simulink model "AdmittanceScanPRBS"  (R2025a)
settings: Solver=VariableStepAuto  StartTime=0.0  StopTime=Tsim  RelTol=1e-3
PreLoadFcn:
  | SimulationTime = 10;
  | AdmittanceScanParameters;
undefined symbols (not defined in the file): Array, Base, BatteryInverter, DiscIntNeverNeededParam, ee_sli_rtmsupport, feeder, fRT, frt, gcbh, GFLBatteryController, GFMBatteryController, gGFM, grid, Grid, line, loadpq, loadstep1, loadstep2, lvrt, LVRT, mGFM, Panel, pll, pmsm, PVController, PVInverter, PVTransformer, scan, time, Ts, VSMbase, windController, windTurbine
libraries: ee_lib x19, eeGeneralControl x17, nesl_utility x16, fl_lib x10, eeTransforms x9, simulink x8, slpidlib x2, batteryecm_lib x1, simulink_extras x1, eePowerMeasurement x1
(part 1 of 4)
settings Model: SimulationMode=accelerator  PacingRate=1.100000  Creator=rajarshd  LastModifiedBy=rajarshd
settings DataIOCC: ReturnWorkspaceOutputsName=Data
settings OptimizationCC: BlockReduction=off  DefaultParameterBehavior=Inlined  BufferReuse=off
settings RTWCC: GPUComputeCapability=3.5

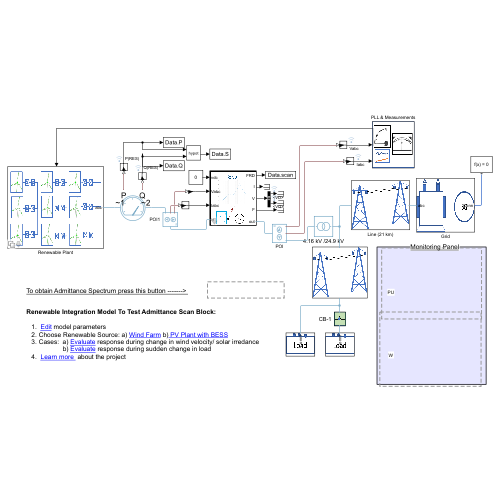
[thumbnail: Simulink's stored preview of the top-level diagram]
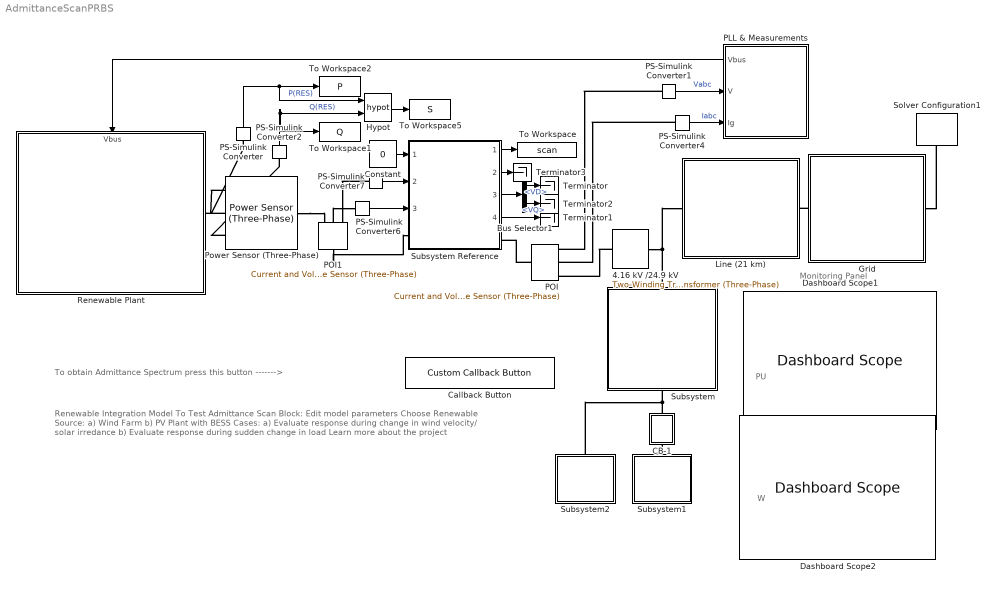
== system AdmittanceScanPRBS ==
  note: W
  note: PU
  note: Monitoring Panel
  note: To obtain Admittance Spectrum press this button ------->
  note: Renewable Integration Model To Test Admittance Scan Block:
      |
      | Edit model parameters
      | Choose Renewable Source: a) Wind Farm b) PV Plant with BESS
      | Cases: a) Evaluate response during change in wind velocity/ solar irredance
      | b) Evaluate response during sudden change in load
      | Learn more about the project
  4.16 kV /24.9 kV : ee_lib/Passive/Transformers/Two-Winding Transformer (Three-Phase)  SRated=PVTransformer.VA A*V  FRated=Grid.frequency Hz  Winding1Connection=ee.enum.windingconnection.Yg  VRated1=PVTransformer.hv V  Winding2Connection=ee.enum.windingconnection.Yg  VRated2=PVTransformer.lv V  CoreType=ee.enum.coretype.threelimb  pu_Rw1=PVTransformer.winding_resistance/2  pu_Rw2=PVTransformer.winding_resistance/2  leakage_reactance_option=ee.enum.transformer_leakage.include  pu_Xl1=PVTransformer.winding_lekage_reactance/2  pu_Xl2=PVTransformer.winding_lekage_reactance/2  magnetizing_resistance_option=ee.enum.transformer_magnetizingResistance.exclude  pu_Rm=500  magnetizing_reactance_option=ee.enum.transformer_magnetizingReactance.exclude  saturation_option=ee.enum.transformer_saturation.exclude  pu_Xm=500  current_data=[0, .002, 1, 2]  magnetic_flux_data=[0, 1.2, 1.5, 1.51]  pu_X0=PVTransformer.zero_sequence_reactance  i1_specify=off  i1_priority=None  i1=[0, 0, 0] A  i1_nominal_specify=off  i1_nominal_value=1  i1_nominal_unit=A  i2_specify=off  i2_priority=None  i2=[0, 0, 0] A  i2_nominal_specify=off  i2_nominal_value=1  i2_nominal_unit=A  phi_specify=off  phi_priority=None  phi=[0, 0, 0]  phi_nominal_specify=off  phi_nominal_value=1  phi_nominal_unit=1  power_dissipated_specify=off  power_dissipated_priority=None  power_dissipated=0 W  power_dissipated_nominal_specify=off  power_dissipated_nominal_value=1  power_dissipated_nominal_unit=W
      settings: InternalSimscapePortConfiguration="{\"Bottom\":[],\"Left\":[{\"id\":\"N1\",\"label\":\"~1\",\"type\":\"foundation.electrical.three_phase\"}],\"Right\":[{\"id\":\"N2\",\"label\":\"~2\",\"type\":\"foundation.electrical.three_phase\"}],\"Top\":[]}"
  Bus Selector1 : BusSelector  OutputSignals=VD,VQ
  CB-1 : Subsystem
      mask Display: image('$imagefile'); % Use "Edit Image" on toolstrip to change.
  Callback Button : CustomCallbackButton  Configuration="{\"components\":[{\"name\":\"BackgroundImageComponent\",\"settings\":{\"image\":{\"size\":[0,0],\"src\":\"default\",\"srcOrientation\":\"Right\"},\"position\":[0,0,1,1]}},{\"name\":\"ButtonStateComponent\",\"settings\":{\"buttonType\":\"latch\",\"clickFcn\":\"Data=sim(bdroot);\\nadmittancescanPRBS(scan.Vd,scan.Vq,scan.Vdc,scan.f,Data.scan,modelorder) \",\"latched\":false,\"offValue\":null,\"onValue\":1,\"position\":[0,0,1,1],\"pressDelay\":\"500\",\"pressFcn\":\"\",\"repeatInterval\":\"0\",\"states\":[{\"horizontalAlignment\":\"center\",\"image\":{\"position\":[0,0,1,1],\"size\":[1,1],\"src\":\"default\",\"srcOrientation\":\"Right\"},\"label\":{\"color\":[1,1,1],\"icon\":{\"size\":[0,0],\"src\":\"default\",\"srcOrientation\":\"Right\"},\"iconOffset\":0,\"iconPlacement\":\"left\",\"opacity\":1,\"show\":true,\"text\":{\"content\":\"Admittance Scan\",\"font\":\"Helvetica\"}},\"labelOffset\":[0,0],\"verticalAlignment\":\"middle\"},{\"horizontalAlignment\":\"center\",\"image\":{\"position\":[0,0,1,1],\"size\":[1,1],\"src\":\"default\",\"srcOrientation\":\"Right\"},\"label\":{\"color\":[0.8509803921568627,0.3254901960784314,0.09803921568627451],\"icon\":{\"size\":[0,0],\"src\":\"default\",\"srcOrientation\":\"Right\"},\"iconOffset\":0,\"iconPlacement\":\"left\",\"opacity\":0,\"show\":true,\"text\":{\"content\":\"Admittance Scan\",\"font\":\"Helvetica\"}},\"labelOffset\":[-0.01428571428571429,-5.551115123125783e-17],\"verticalAlignment\":\"middle\"},{\"horizontalAlignment\":\"center\",\"image\":{\"position\":[0,0,1,1],\"size\":[1,1],\"src\":\"default\",\"srcOrientation\":\"Right\"},\"label\":{\"color\":[0.01176470588,0.01176470588,0.01176470588,1],\"icon\":{\"size\":[0,0],\"src\":\"default\",\"srcOrientation\":\"Right\"},\"iconOffset\":0,\"iconPlacement\":\"left\",\"opacity\":1,\"show\":true,\"text\":{\"content\":\"Admittance Scan\",\"font\":\"Helvetica\"}},\"labelOffset\":[0,0],\"verticalAlignment\":\"middle\"},{\"horizontalAlignment\":\"center\",\"image\":{\"position\":[0,0,1,1],\"size\":[1,1],\"src\":\"default\",\"srcOrientation\":\"Right\"},\"label\":{\"color\":[0.01176470588,0.01176470588,0.01176470588,1],\"icon\":{\"size\":[0,0],\"src\":\"default\",\"srcOrientation\":\"Right\"},\"iconOffset\":0,\"iconPlacement\":\"left\",\"opacity\":1,\"show\":true,\"text\":{\"content\":\"Admittance Scan\",\"font\":\"Helvetica\"}},\"labelOffset\":[0,0],\"verticalAlignment\":\"middle\"}]}},{\"name\":\"ForegroundImageComponent\",\"settings\":{\"image\":{\"size\":[0,0],\"src\":\"default\",\"srcOrientation\":\"Right\"},\"isForeground\":1,\"position\":[0,0,1,1]}}],\"derived\":{\"blockParameters\":{\"AutoActivate\":true,\"ButtonText\":\"Admittance Scan\",\"ButtonType\":\"Latch\",\"ClickFcn\":\"Data=sim(bdroot);\\nadmittancescanPRBS(scan.Vd,scan.Vq,scan.Vdc,scan.f,Data.scan,modelorder) \",\"OnValue\":1,\"PressDelay\":\"500\",\"PressFcn\":\"\",\"RepeatInterval\":\"0\",\"fixedAspectRatio\":\"off\"}},\"settings\":{\"BindingType\":\"standalone\",\"autoActivate\":true,\"backgroundColor\":[244,244,244,1],\"backgroundOffset\":0.2,\"backgroundOpacity\":1,\"fixedAspectRatio\":\"off\",\"foregroundColor\":[0.01176470588,0.01176470588,0.01176470588,1],\"migratedFromLegacy\":true,\"useBackgroundColor\":true,\"variant\":\"callback\",\"version\":\"R2025a\"},\"type\":\"Button\"}"  CustomBackgroundColor="{\"color\":[0,0.4470588235294118,0.7411764705882353],\"show\":true}"
  Constant : Constant  Value=0
  Dashboard Scope1 : DashboardScope  Ymin=0  Ymax=5e7  FontColor=[0.0, 0.0, 0.0]
  Dashboard Scope2 : DashboardScope  Ymin=-0.1  Ymax=1.5  FontColor=[0.0, 0.0, 0.0]
  Grid : Subsystem  VariantControl=Voltage Source
      mask Display: image('grid.png');
  Hypot : Math  Operator=hypot
  Line (21 km) : Subsystem
      mask Display: image('Network.png');
  PLL & Measurements : Subsystem
      settings: PortSchema="{\"entries\":[{\"content\":{\"sides\":[{\"content\":{\"connectorIds\":[\"Out1\",\"In1\",\"In2\"]},\"type\":\"ConnectorPlacement.EquallySpacedRectSide\",\"uuid\":\"76485780-20fe-4fcf-8224-69648da6ed2a\"},{\"content\":{\"side\":\"RIGHT\"},\"type\":\"ConnectorPlacement.EquallySpacedRectSide\",\"uuid\":\"f19a6390-e634-42c7-8d46-4cd80cbab182\"},{\"content\":{\"side\":\"TOP\"},\"type\":\"ConnectorPlacement.EquallySpacedRectSide\",\"uuid\":\"87682f72-1844-428e-be70-ad7ca3191ee3\"}]},\"type\":\"ConnectorPlacement.EquallySpacedConnector\",\"uuid\":\"f2136b07-48ec-402b-adb3-18c0bac2157c\"}],\"packageUris\":[\"http://schema.mathworks.com/mf0/Connector/R2020b\"],\"version\":\"1.0\"}"
      mask Display: image('measurements.png'); % Use "Edit Image" on toolstrip to change.
  POI : ee_lib/Sensors & Transducers/Current and Voltage Sensor (Three-Phase)  vMeasurementType=ee.enum.vmeasurement.lg  outputUnit=ee.enum.unit.pu  SRated=base.mVA A*V  VRated=base.kV V  I_specify=off  I_priority=None  I=[0, 0, 0] A  I_nominal_specify=off  I_nominal_value=1  I_nominal_unit=A  V_specify=off  V_priority=None  V=[0, 0, 0] V  V_nominal_specify=off  V_nominal_value=1  V_nominal_unit=V
      settings: InternalSimscapePortConfiguration="{\"Bottom\":[],\"Left\":[{\"id\":\"N1\",\"label\":\"~1\",\"type\":\"foundation.electrical.three_phase\"}],\"Right\":[{\"id\":\"V_output\",\"label\":\"V\",\"type\":\"output\"},{\"id\":\"I_output\",\"label\":\"I\",\"type\":\"output\"},{\"id\":\"N2\",\"label\":\"~2\",\"type\":\"foundation.electrical.three_phase\"}],\"Top\":[]}"
  POI1 : ee_lib/Sensors & Transducers/Current and Voltage Sensor (Three-Phase)  vMeasurementType=ee.enum.vmeasurement.ll  outputUnit=ee.enum.unit.si  SRated=base.mVA A*V  VRated=base.kV V  I_specify=off  I_priority=None  I=[0, 0, 0] A  I_nominal_specify=off  I_nominal_value=1  I_nominal_unit=A  V_specify=off  V_priority=None  V=[0, 0, 0] V  V_nominal_specify=off  V_nominal_value=1  V_nominal_unit=V
      settings: InternalSimscapePortConfiguration="{\"Bottom\":[],\"Left\":[{\"id\":\"N1\",\"label\":\"~1\",\"type\":\"foundation.electrical.three_phase\"}],\"Right\":[{\"id\":\"V_output\",\"label\":\"V\",\"type\":\"output\"},{\"id\":\"I_output\",\"label\":\"I\",\"type\":\"output\"},{\"id\":\"N2\",\"label\":\"~2\",\"type\":\"foundation.electrical.three_phase\"}],\"Top\":[]}"
  PS-Simulink Converter{,1..2,4,6..7} (6 alike) : nesl_utility/PS-Simulink Converter  PhysicalDomain=network_engine_domain  SubClassName=ps_output  LeftPortType=input  RightPortType=output  PseudoPeriodic=off  Frequencies=[]  VectorFormat=inherit  Unit=inherit  AffineConversion=off
  Power Sensor (Three-Phase) : ee_lib/Sensors & Transducers/Power Sensor (Three-Phase)  load_type=ee.enum.passive.type_balanced.balanced  f0=60 Hz  config=ee.enum.with_neutral.no  rho=1
      settings: InternalSimscapePortConfiguration="{\"Bottom\":[],\"Left\":[{\"id\":\"N1\",\"label\":\"~1\",\"type\":\"foundation.electrical.three_phase\"}],\"Right\":[{\"id\":\"N2\",\"label\":\"~2\",\"type\":\"foundation.electrical.three_phase\"}],\"Top\":[{\"id\":\"Pm\",\"label\":\"P\",\"type\":\"output\"},{\"id\":\"Qm\",\"label\":\"Q\",\"type\":\"output\"}]}"
  Renewable Plant : Subsystem  Variant=on  mask{Choice=Wind Farm, Control=VSM Using Turbine Inertia, LabelModeActiveChoice1=BESSGridSupporting, nGFL=4, nGFM=0}
      mask prompts: Choice "Renewable Plant Model"; Control "GFM Controller"; LabelModeActiveChoice1 "Choose BESS Controller"; nGFL "Number of GFL Wind Generators"; nGFM "Number of GFM Wind Turbines"
      settings: PortSchema="{\"entries\":[{\"content\":{\"sides\":[{\"content\":{},\"type\":\"ConnectorPlacement.EquallySpacedRectSide\",\"uuid\":\"4ca8547f-3459-43d1-a89a-15dca644f6a7\"},{\"content\":{\"connectorIds\":[\"RConn1\"],\"side\":\"RIGHT\"},\"type\":\"ConnectorPlacement.EquallySpacedRectSide\",\"uuid\":\"f647f9d8-3ccd-4429-b3c9-fe10a5d661de\"},{\"content\":{\"connectorIds\":[\"In1\"],\"side\":\"TOP\"},\"type\":\"ConnectorPlacement.EquallySpacedRectSide\",\"uuid\":\"1b35996a-53e0-4772-8d84-1134ddf5dd6b\"}]},\"type\":\"ConnectorPlacement.EquallySpacedConnector\",\"uuid\":\"b195f748-0d0d-4b03-b11c-4c7a353756a0\"}],\"packageUris\":[\"http://schema.mathworks.com/mf0/Connector/R2020b\"],\"version\":\"1.0\"}"
      mask TypeOptions Choice: PV Plant | Wind Farm
      mask Callback Choice:
      | h = Simulink.Mask.get(gcb);
      | Choice = get_param(gcb,'Choice');
      | switch Choice
      |     case 'Wind Farm'
      |         h.Parameters(find(string({h.Parameters.Name}) == 'nGFL')).Visible = 'on';
      |         h.Parameters(find(string({h.Parameters.Name}) == 'nGFM')).Visible = 'on';
      |         h.Parameters(find(string({h.Parameters.Name}) == 'LabelModeActiveChoice1')).Visible = 'off';
      |         h.Parameters(find(string({h.Parameters.Name}) == 'Control')).Visible = 'on';
      |     case 'PV Plant'
      |         h.Parameters(find(string({h.Parameters.Name}) == 'nGFL')).Visible = 'off';
      |         h.Parameters(find(string({h.Parameters.Name}) == 'nGFM')).Visible = 'off';
      |         h.Parameters(find(string({h.Parameters.Name}) == 'LabelModeActiveChoice1')).Visible = 'on';
      |         h.Parameters(find(string({h.Parameters.Name}) == 'Control')).Visible = 'off';
      | end
      mask TypeOptions Control: Wind Farm/Control
      mask TypeOptions LabelModeActiveChoice1: PV Plant/LabelModeActiveChoice1
      mask TypeOptions nGFL: Wind Farm/nGFL
      mask TypeOptions nGFM: Wind Farm/nGFM
      mask DialogControl Container4 Prompt: Plant Specifications
  Solver Configuration1 : nesl_utility/Solver Configuration  PhysicalDomain=network_engine_domain  SubClassName=solver  LeftPortType=input  RightPortType=generic  Tones=[]  Harmonics=[]  SimulateNoise=off  Profile=off  UseLocalSampling=off  EnableSwitchedLinearOptims=on  FrequencyDomain=off  UseCCode=off  RelTol=0.001  AbsTol=1e-06  MinStep=1e-09  ToWorkspace=off  RevertToSquareIcSolve=off  NumHomotopyIterations=100  PhasorMode=off  PhasorModeNumHarmonics=1  ConsistencySolver=NEWTON_XTOL_AFTER_FTOL  IndexReductionMethod=None  DoDC=off  ResidualTolerance=1e3  ConsistencyTolSource=GLOBAL  ConsistencyAbsTol=0.001  ConsistencyRelTol=0.001  ConsistencyTolFactor=0.001  UseLocalSolver=on  LocalSolverChoice=NE_BACKWARD_EULER_ADVANCER  ResolveIndetEquations=off  FunctionEvalNumThread=1  LocalSolverSampleTime=5e-5  DoFixedCost=on  MaxNonlinIter=1  MaxModeIter=2  ComputeImpulses=off  ImpulseIterations=2  LinearAlgebra=Sparse  LinearAlgebraNumThread=0  EquationFormulation=NE_TIME_EF  DelaysMemoryBudget=1024  AutomaticFiltering=on  FilteringTimeConstant=0.001  PartitionStorageMethod=AS_NEEDED  PartitionMemoryBudget=1024  PartitionMethod=ROBUST  MultibodyUseLocalSolver=off  MultibodyLocalSolverChoice=ODE1  MultibodyLocalSolverSampleTime=0.001
  Subsystem : Subsystem
      mask Display: image('Network.png');
  Subsystem Reference : Subsystem  ReferencedSubsystem=ScanBlockwithDC  F0=grid.frequency  Theta0=0  Kp_LF=pll.kp  Ki_LF=pll.ki  Ts=Ts  voltage=Base.KV_base_new  voltagedc=0  mva=Base.MVA_base_new  Amplitude=scan.Vd  Amplitude1=scan.Vq  Amplitudedc=0  f=scan.f  T=1/scan.samplingfrequency  Tdis=scan.start  Tend=scan.end  VSelect=Equivalent Series Voltage (V)  Hold=Yes
  Subsystem1 : Subsystem
      mask Display: image('Load.png');
  Subsystem2 : Subsystem
      mask Display: image('Load.png');
  Terminator{,1..3} (4 alike) : Terminator
  To Workspace : ToWorkspace  VariableName=scan  SaveFormat=Timeseries  SampleTime=-1
  To Workspace1 : ToWorkspace  VariableName=Q  SaveFormat=Timeseries  SampleTime=1/5e3
      settings: Save2DSignal=2-D array (concatenate along first dimension)
  To Workspace2 : ToWorkspace  VariableName=P  SaveFormat=Timeseries  SampleTime=1/5e3
      settings: Save2DSignal=2-D array (concatenate along first dimension)
  To Workspace5 : ToWorkspace  VariableName=S  SaveFormat=Timeseries  SampleTime=1/5e3
      settings: Save2DSignal=2-D array (concatenate along first dimension)
  wires:
  PS-Simulink Converter4/1 -> PLL & Measurements/2(Ig)  "Iabc"
  PS-Simulink Converter1/1 -> PLL & Measurements/1(V)  "Vabc"
  PLL & Measurements/1(Vbus) -> Renewable Plant/1(Vbus)
  Hypot/1 -> To Workspace5/1
  PS-Simulink Converter2/1 -> To Workspace1/1, Hypot/2  "Q(RES)"
  PS-Simulink Converter/1 -> Hypot/1, To Workspace2/1  "P(RES)"
  PS-Simulink Converter6/1 -> Subsystem Reference/3
  PS-Simulink Converter7/1 -> Subsystem Reference/2
  Subsystem Reference/4 -> Terminator1/1
  Bus Selector1/1 -> Terminator/1  "<VD>"
  Bus Selector1/2 -> Terminator2/1  "<VQ>"
  Subsystem Reference/1 -> To Workspace/1
  Subsystem Reference/3 -> Bus Selector1/1
  Subsystem Reference/2 -> Terminator3/1
  Constant/1 -> Subsystem Reference/1
  connections:
  Power Sensor (Three-Phase)/LConn3 -- PS-Simulink Converter2/LConn1
  Power Sensor (Three-Phase)/LConn2 -- PS-Simulink Converter/LConn1
  PS-Simulink Converter1/LConn1 -- POI/RConn1
  PS-Simulink Converter4/LConn1 -- POI/RConn2
  Grid/LConn1 -- Line (21 km)/RConn1
  Subsystem/LConn1 -- Line (21 km)/LConn1 -- 4.16 kV /24.9 kV/LConn1
  Subsystem1/LConn1 -- CB-1/RConn1
  4.16 kV /24.9 kV/RConn1 -- POI/RConn3
  Grid/RConn1 -- Solver Configuration1/RConn1
  POI/LConn1 -- Subsystem Reference/RConn1
  Power Sensor (Three-Phase)/LConn1 -- Renewable Plant/RConn1
  POI1/LConn1 -- Subsystem Reference/LConn1
  POI1/RConn2 -- PS-Simulink Converter6/LConn1
  PS-Simulink Converter7/LConn1 -- POI1/RConn1
  Power Sensor (Three-Phase)/RConn1 -- POI1/RConn3
  CB-1/LConn1 -- Subsystem2/LConn1 -- Subsystem/RConn1

== system AdmittanceScanPRBS/CB-1 ==
  Circuit Breaker Step off3 : ee_lib/Switches & Breakers/Circuit Breaker (Three-Phase)  R_closed=0.001 Ohm  G_open=1e-4 1/Ohm  threshold=0.5 V  breaker_behavior=ee.enum.switches.breakerBehavior.zeroCrossingEnable
      settings: InternalSimscapePortConfiguration="{\"Bottom\":[],\"Left\":[{\"id\":\"vT\",\"label\":\"vT\",\"type\":\"input\"},{\"id\":\"N1\",\"label\":\"~1\",\"type\":\"foundation.electrical.three_phase\"}],\"Right\":[{\"id\":\"N2\",\"label\":\"~2\",\"type\":\"foundation.electrical.three_phase\"}],\"Top\":[]}"
  Simulink-PS Converter3 : nesl_utility/Simulink-PS Converter  PhysicalDomain=network_engine_domain  SubClassName=ps_input  LeftPortType=input  RightPortType=output  PseudoPeriodic=off  Frequencies=[]  NoiseDistribution=none  NoiseParameters=[]  Unit=1  AffineConversion=off  FilteringAndDerivatives=zero  SimscapeFilterOrder=1  InputFilterTimeConstant=0.001  UdotUserProvided=1
  Step off3 : Step  Time=time.loadswitch  Before=loadstep1  After=loadstep2  SampleTime=Ts
  Conn2 : PMIOPort  Side=Left
  Conn1 : PMIOPort  Port=2  Side=Right
  wires:
  Step off3/1 -> Simulink-PS Converter3/1
  connections:
  Circuit Breaker Step off3/LConn2 -- Conn2/RConn1
  Circuit Breaker Step off3/LConn1 -- Simulink-PS Converter3/RConn1
  Circuit Breaker Step off3/RConn1 -- Conn1/RConn1

== system AdmittanceScanPRBS/Grid ==
  Electrical Reference : fl_lib/Electrical/Electrical Elements/Electrical Reference
  Voltage Source (Three-Phase) : ee_lib/Sources/Voltage Source (Three-Phase)  vline_rms=24.9e3 V  shift=0 deg  freq=60 Hz  impedance_option=0  SShortCircuit=1e6 A*V  XR=15  R=0.01 Ohm  L=3.97e-4 H  harmonic_option=0  harmonic_orders=[5, 7, 11, 13]  harmonic_ratios=[.1, .1, .1, .1]  G_parasitic=0 1/Ohm  I_specify=off  I_priority=None  I=[0, 0, 0] A  I_nominal_specify=off  I_nominal_value=1  I_nominal_unit=A
  abc : PMIOPort  Side=Left
  Conn : PMIOPort  Port=2  Side=Right
  connections:
  Voltage Source (Three-Phase)/RConn1 -- abc/RConn1
  Conn/RConn1 -- Electrical Reference/LConn1 -- Voltage Source (Three-Phase)/LConn1

== system AdmittanceScanPRBS/Line (21 km) ==
  Electrical Reference : fl_lib/Electrical/Electrical Elements/Electrical Reference
  Electrical Reference1 : fl_lib/Electrical/Electrical Elements/Electrical Reference
  Transmission Line (Three-Phase) : ee_lib/Passive/Lines/Transmission Line (Three-Phase)  length=line.length1 km  freq=grid.frequency Hz  R=line.r Ohm/km  L=line.l mH/km  M=line.m mH/km  Cl=line.cll uF/km  Cg=line.clg uF/km  Rm=0 Ohm/km  ModelTwoSections=ee.enum.enable.no  N=1  InterfacePosition=0.5 km  N1sec=1  N2sec=1  Access_ground=ee.enum.enable.no  R_parasitic=1e-9 Ohm  G_parasitic=1e-9 1/Ohm
      settings: InternalSimscapePortConfiguration="{\"Bottom\":[],\"Left\":[{\"id\":\"N1\",\"label\":\"~1\",\"type\":\"foundation.electrical.three_phase\"},{\"id\":\"g1\",\"label\":\"g1\",\"type\":\"foundation.electrical.electrical\"}],\"Right\":[{\"id\":\"N2\",\"label\":\"~2\",\"type\":\"foundation.electrical.three_phase\"},{\"id\":\"g2\",\"label\":\"g2\",\"type\":\"foundation.electrical.electrical\"}],\"Top\":[]}"
  Conn1 : PMIOPort  Side=Right
  Conn2 : PMIOPort  Port=2  Side=Left
  connections:
  Electrical Reference/LConn1 -- Transmission Line (Three-Phase)/RConn2
  Electrical Reference1/LConn1 -- Transmission Line (Three-Phase)/LConn2
  Conn1/RConn1 -- Transmission Line (Three-Phase)/RConn1
  Conn2/RConn1 -- Transmission Line (Three-Phase)/LConn1

== system AdmittanceScanPRBS/PLL & Measurements ==
  V : Inport
  Ig : Inport  Port=2
  Measurement1 : Subsystem
  Measurement2 : Subsystem
  PLL : Subsystem
  Out Bus Element : Outport  PortName=Vbus  Element=Vq
  Out Bus Element1 : Outport  PortName=Vbus  Element=Vd
  Out Bus Element2 : Outport  PortName=Vbus  Element=w
  Out Bus Element3 : Outport  PortName=Vbus  Element=Theta
  Out Bus Element4 : Outport  PortName=Vbus  Element=Vmag
  Out Bus Element5 : Outport  PortName=Vbus  Element=Id
  Out Bus Element6 : Outport  PortName=Vbus  Element=Iq
  wires:
  V/1 -> Measurement2/1(u)
  PLL/2(freq) -> Out Bus Element2/1  "w"
  PLL/5(Vq) -> Out Bus Element/1  "Vq"
  PLL/3(angle) -> Out Bus Element3/1
  PLL/4(Vd) -> Out Bus Element1/1  "Vd"
  Measurement2/1(Vg) -> PLL/1(abc)
  PLL/1(mag) -> Out Bus Element4/1  "Vmag"
  Measurement1/1(Ig) -> PLL/2(Ig)
  Ig/1 -> Measurement1/1(u)
  PLL/7(Iq) -> Out Bus Element6/1  "Iq"
  PLL/6(Id) -> Out Bus Element5/1  "Id"

== system AdmittanceScanPRBS/Renewable Plant ==
  Vbus : Inport
  PV Plant : Subsystem  VariantControl=Choice==1  mask{LabelModeActiveChoice1=BESSGridSupporting}
      mask prompts: LabelModeActiveChoice1 "Choose BESS Controller"
      mask TypeOptions LabelModeActiveChoice1: 60 MWhr Battery Energy Storage/LabelModeActiveChoice1
      mask Display: image('PV_park.png');
  Wind Farm : Subsystem  VariantControl=Choice==2  mask{nGFL=4, nGFM=0, Control=VSM Using Turbine Inertia}
      mask prompts: nGFL "Number of GFL Wind Generators"; nGFM "Number of GFM Wind Turbines"; Control "GFM Controller"
      mask TypeOptions nGFL: 1 | 2 | 3 | 4 | 5 | 6 | 7
      mask Callback nGFL:
      | choice=get_param(gcb,'nGFL');
      |   switch choice
      |     case '1'
      |          set_param(strcat(gcb,'/Wind Turbine 1(GFL) 1'),'Commented','on');
      |          set_param(strcat(gcb,'/Wind Turbine 1(GFL) 2'),'Commented','on');
      |          set_param(strcat(gcb,'/Wind Turbine 1(GFL) 3'),'Commented','on');
      |          set_param(strcat(gcb,'/Wind Turbine 1(GFL) 4'),'Commented','on');
      |          set_param(strcat(gcb,'/Wind Turbine 1(GFL) 5'),'Commented','on');
      |          set_param(strcat(gcb,'/Wind Turbine 1(GFL) 6'),'Commented','on');
      |          set_param(strcat(gcb,'/Wind Turbine 1(GFL) '),'Commented','off');
      |     case '2'
      |          set_param(strcat(gcb,'/Wind Turbine 1(GFL) 1'),'Commented','on');
      |          set_param(strcat(gcb,'/Wind Turbine 1(GFL) 2'),'Commented','off');
      |          set_param(strcat(gcb,'/Wind Turbine 1(GFL) 3'),'Commented','on');
      |          set_param(strcat(gcb,'/Wind Turbine 1(GFL) 4'),'Commented','on');
      |          set_param(strcat(gcb,'/Wind Turbine 1(GFL) 5'),'Commented','on');
      |          set_param(strcat(gcb,'/Wind Turbine 1(GFL) 6'),'Commented','on');
      |          set_param(strcat(gcb,'/Wind Turbine 1(GFL) '),'Commented','off');
      |     case '3'
      |          set_param(strcat(gcb,'/Wind Turbine 1(GFL) 1'),'Commented','off');
      |          set_param(strcat(gcb,'/Wind Turbine 1(GFL) 2'),'Commented','off');
      |          set_param(strcat(gcb,'/Wind Turbine 1(GFL) 3'),'Commented','on');
      |          set_param(strcat(gcb,'/Wind Turbine 1(GFL) 4'),'Commented','on');
      |          set_param(strcat(gcb,'/Wind Turbine 1(GFL) 5'),'Commented','on');
      |          set_param(strcat(gcb,'/Wind Turbine 1(GFL) 6'),'Commented','on');
      |          set_param(strcat(gcb,'/Wind Turbine 1(GFL) '),'Commented','off');
      |     case '4'
      |          set_param(strcat(gcb,'/Wind Turbine 1(GFL) 1'),'Commented','off');
      |          set_param(strcat(gcb,'/Wind Turbine 1(GFL) 2'),'Commented','off');
      |          set_param(strcat(gcb,'/Wind Turbine 1(GFL) 3'),'Commented','off');
      |          set_param(strcat(gcb,'/Wind Turbine 1(GFL) 4'),'Commented','on');
      |          set_param(strcat(gcb,'/Wind Turbine 1(GFL) 5'),'Commented','on');
      |          set_param(strcat(gcb,'/Wind Turbine 1(GFL) 6'),'Commented','on');
      |          set_param(strcat(gcb,'/Wind Turbine 1(GFL) '),'Commented','off');
      |     case '5'
      |          set_param(strcat(gcb,'/Wind Turbine 1(GFL) 1'),'Commented','off');
      |          set_param(strcat(gcb,'/Wind Turbine 1(GFL) 2'),'Commented','off');
      |          set_param(strcat(gcb,'/Wind Turbine 1(GFL) 3'),'Commented','off');
      |          set_param(strcat(gcb,'/Wind Turbine 1(GFL) 4'),'Commented','off');
      |          set_param(strcat(gcb,'/Wind Turbine 1(GFL) 5'),'Commented','on');
      |          set_param(strcat(gcb,'/Wind Turbine 1(GFL) 6'),'Commented','on');
      |          set_param(strcat(gcb,'/Wind Turbine 1(GFL) '),'Commented','off');
      |     case '6'
      |          set_param(strcat(gcb,'/Wind Turbine 1(GFL) 1'),'Commented','off');
      |          set_param(strcat(gcb,'/Wind Turbine 1(GFL) 2'),'Commented','off');
      |          set_param(strcat(gcb,'/Wind Turbine 1(GFL) 3'),'Commented','off');
      |          set_param(strcat(gcb,'/Wind Turbine 1(GFL) 4'),'Commented','off');
      |          set_param(strcat(gcb,'/Wind Turbine 1(GFL) 5'),'Commented','off');
      |          set_param(strcat(gcb,'/Wind Turbine 1(GFL) 6'),'Commented','on');
      |          set_param(strcat(gcb,'/Wind Turbine 1(GFL) '),'Commented','off');
      |     case '7'
      |          set_param(strcat(gcb,'/Wind Turbine 1(GFL) 1'),'Commented','off');
      |          set_param(strcat(gcb,'/Wind Turbine 1(GFL) 2'),'Commented','off');
      |          set_param(strcat(gcb,'/Wind Turbine 1(GFL) 3'),'Commented','off');
      |          set_param(strcat(gcb,'/Wind Turbine 1(GFL) 4'),'Commented','off');
      |          set_param(strcat(gcb,'/Wind Turbine 1(GFL) 5'),'Commented','off');
      |          set_param(strcat(gcb,'/Wind Turbine 1(GFL) 6'),'Commented','off');
      |          set_param(strcat(gcb,'/Wind Turbine 1(GFL) '),'Commented','off');
      | end
      mask TypeOptions nGFM: 0 | 1 | 2
      mask Callback nGFM:
      | choice=get_param(gcb,'nGFM');
      |   switch choice
      |     case '0'
      |          set_param(strcat(gcb,'/Wind Turbine (GFM)'),'Commented','on');
      |          set_param(strcat(gcb,'/Wind Turbine (GFM)1'),'Commented','on');
      |          set_param(strcat(gcb,'/Measurements1'),'Commented','on');
      |          set_param(strcat(gcb,'/Collector Line7'),'Commented','on');
      |          set_param(strcat(gcb,'/Collector Line5'),'Commented','on');
      |          set_param(strcat(gcb,'/Bus Selector2'),'Commented','on');
      |     case '1'
      |          set_param(strcat(gcb,'/Wind Turbine (GFM)'),'Commented','on');
      |          set_param(strcat(gcb,'/Wind Turbine (GFM)1'),'Commented','off');
      |          set_param(strcat(gcb,'/Measurements1'),'Commented','off');
      |          set_param(strcat(gcb,'/Collector Line5'),'Commented','on');
      |          set_param(strcat(gcb,'/Collector Line7'),'Commented','off');
      |          set_param(strcat(gcb,'/Bus Selector2'),'Commented','on');
      |     case '2'
      |          set_param(strcat(gcb,'/Wind Turbine (GFM)'),'Commented','off');
      |          set_param(strcat(gcb,'/Wind Turbine (GFM)1'),'Commented','off');
      |          set_param(strcat(gcb,'/Measurements1'),'Commented','off');
      |          set_param(strcat(gcb,'/Collector Line5'),'Commented','off');
      |          set_param(strcat(gcb,'/Collector Line7'),'Commented','off');
      |          set_param(strcat(gcb,'/Bus Selector2'),'Commented','off');
      |   end
      mask TypeOptions Control: Wind Turbine (GFM)/Control | Wind Turbine (GFM)1/Control
      mask DialogControl Control1 Prompt: This is a Wind Farm with type-4 GFL and GFM Wind Turbine Generators
      mask Display: image('WindFarmModel.PNG');
  abc : PMIOPort  Side=Right

== system AdmittanceScanPRBS/Subsystem ==
  Electrical Reference : fl_lib/Electrical/Electrical Elements/Electrical Reference
  Electrical Reference1 : fl_lib/Electrical/Electrical Elements/Electrical Reference
  Transmission Line (Three-Phase) : ee_lib/Passive/Lines/Transmission Line (Three-Phase)  length=line.length2 km  freq=grid.frequency Hz  R=line.r Ohm/km  L=line.l mH/km  M=line.m mH/km  Cl=line.cll uF/km  Cg=line.clg uF/km  Rm=0 Ohm/km  ModelTwoSections=ee.enum.enable.no  N=1  InterfacePosition=0.5 km  N1sec=1  N2sec=1  Access_ground=ee.enum.enable.no  R_parasitic=1e-9 Ohm  G_parasitic=1e-9 1/Ohm
      settings: InternalSimscapePortConfiguration="{\"Bottom\":[],\"Left\":[{\"id\":\"N1\",\"label\":\"~1\",\"type\":\"foundation.electrical.three_phase\"},{\"id\":\"g1\",\"label\":\"g1\",\"type\":\"foundation.electrical.electrical\"}],\"Right\":[{\"id\":\"N2\",\"label\":\"~2\",\"type\":\"foundation.electrical.three_phase\"},{\"id\":\"g2\",\"label\":\"g2\",\"type\":\"foundation.electrical.electrical\"}],\"Top\":[]}"
  Conn1 : PMIOPort  Side=Left
  Conn2 : PMIOPort  Port=2  Side=Right
  connections:
  Electrical Reference/LConn1 -- Transmission Line (Three-Phase)/RConn2
  Electrical Reference1/LConn1 -- Transmission Line (Three-Phase)/LConn2
  Conn1/RConn1 -- Transmission Line (Three-Phase)/LConn1
  Conn2/RConn1 -- Transmission Line (Three-Phase)/RConn1

== system AdmittanceScanPRBS/Subsystem1 ==
  Electrical Reference1 : fl_lib/Electrical/Electrical Elements/Electrical Reference
  Wye-Connected Load : ee_lib/Passive/RLC Assemblies/Wye-Connected Load  port_option=ee.enum.threePhasePort.composite  parameterization=ee.enum.rlc.parameterization.ratedpower  component_structure=ee.enum.rlc.structure.R  component_structure_PQ=ee.enum.rlc.structure.SeriesRL  R=1 Ohm  L=1e-3 H  C=1e-6 F  VRated=24e3 V  FRated=60 Hz  P=loadpq.P*0.2 MW  Qpos=loadpq.Q*0.2 A*V  Qneg=-1e2 A*V  R_parasitic=0 Ohm  G_parasitic=0 1/Ohm  R_parasitic_PQ=0 Ohm  G_parasitic_PQ=0 1/Ohm  Vmag0=24e3 V  Vang0=0 deg  Freq0=60 Hz  IL_specify=off  IL_priority=High  IL=[0, 0, 0] A  IL_nominal_specify=off  IL_nominal_value=1  IL_nominal_unit=A  VC_specify=off  VC_priority=High  VC=[0, 0, 0] V  VC_nominal_specify=off  VC_nominal_value=1  VC_nominal_unit=V
  Conn1 : PMIOPort  Side=Left
  connections:
  Electrical Reference1/LConn1 -- Wye-Connected Load/RConn1
  Wye-Connected Load/LConn1 -- Conn1/RConn1

== system AdmittanceScanPRBS/Subsystem2 ==
  Electrical Reference1 : fl_lib/Electrical/Electrical Elements/Electrical Reference
  Wye-Connected Load : ee_lib/Passive/RLC Assemblies/Wye-Connected Load  port_option=ee.enum.threePhasePort.composite  parameterization=ee.enum.rlc.parameterization.ratedpower  component_structure=ee.enum.rlc.structure.R  component_structure_PQ=ee.enum.rlc.structure.SeriesRL  R=1 Ohm  L=1e-3 H  C=1e-6 F  VRated=24e3 V  FRated=60 Hz  P=loadpq.P*0.8 MW  Qpos=loadpq.Q*0.8 A*V  Qneg=-1e2 A*V  R_parasitic=0 Ohm  G_parasitic=0 1/Ohm  R_parasitic_PQ=0 Ohm  G_parasitic_PQ=0 1/Ohm  Vmag0=24e3 V  Vang0=0 deg  Freq0=60 Hz  IL_specify=off  IL_priority=High  IL=[0, 0, 0] A  IL_nominal_specify=off  IL_nominal_value=1  IL_nominal_unit=A  VC_specify=off  VC_priority=High  VC=[0, 0, 0] V  VC_nominal_specify=off  VC_nominal_value=1  VC_nominal_unit=V
  Conn1 : PMIOPort  Side=Left
  connections:
  Electrical Reference1/LConn1 -- Wye-Connected Load/RConn1
  Wye-Connected Load/LConn1 -- Conn1/RConn1

== system AdmittanceScanPRBS/PLL & Measurements/Measurement1 ==
  u : Inport
  Ig : Outport
  wires:
  u/1 -> Ig/1

== system AdmittanceScanPRBS/PLL & Measurements/Measurement2 ==
  u : Inport
  Vg : Outport
  wires:
  u/1 -> Vg/1

== system AdmittanceScanPRBS/PLL & Measurements/PLL ==
  abc : Inport
  Ig : Inport  Port=2
  Demux : Demux  Outputs=3
  Demux1 : Demux  Outputs=3
  Park Transform : eeTransforms/Park Transform  AxisAlignment=Q-axis  PowerInvariant=off
  Park Transform1 : eeTransforms/Park Transform  AxisAlignment=Q-axis  PowerInvariant=off
  "Sinusoidal Measurement (PLL, Three-Phase)1" : Subsystem  LoadFcn=ee_sli_rtmsupport( 'loadfcn', gcbh );  mask(Sinusoidal Measurement (PLL, Three-Phase)){Kp_LF=pll.kp, Ki_LF=pll.ki*0.25, F0=grid.frequency, Theta0=0, Ts=Ts}
      mask prompts: Kp_LF "physmod:ee:library:comments:control:eeSinusoidalMeasurement:LoopFilterProportionalGain_MP"; Ki_LF "physmod:ee:library:comments:control:eeSinusoidalMeasurement:LoopFilterIntegralGain_MP"; F0 "physmod:ee:library:comments:control:eeSinusoidalMeasurement:InitialFrequencyHz_MP"; Theta0 "physmod:ee:library:comments:control:eeSinusoidalMeasurement:InitialPhaseAnglerad_MP"; Ts "physmod:ee:library:comments:control:eeSinusoidalMeasurement:SampleTime1ForInherited_MP"
      mask help: physmod:ee:library:comments:control:eeSinusoidalMeasurement:SinusoidalPowerMeasurementPLLThreePhase_MD
      mask init:
      | timeDomain = ee.mask.initializeThreePhaseSinusoidalMeasurementPLL(Ts);
      settings: CopyFcn=ee_sli_rtmsupport( 'copyfcn', gcbh );  DeleteFcn=ee_sli_rtmsupport( 'deletefcn', gcbh );  ModelCloseFcn=ee_sli_rtmsupport( 'modelclosefcn', gcbh );  PostSaveFcn=ee_sli_rtmsupport( 'postsavefcn', gcbh );  PreCopyFcn=ee_sli_rtmsupport( 'precopyfcn', gcbh );  OpenFcn=ee_sli_rtmsupport( 'openfcn', gcbh );  CloseFcn=ee_sli_rtmsupport( 'closefcn', gcbh );  PreDeleteFcn=ee_sli_rtmsupport( 'predeletefcn', gcbh );
      settings: LibrarySourceBlock=|
      | ee_sl_lib/Measurements/Sinusoidal Measurement
      | (PLL, Three-Phase)
      mask Help: web(nesl_help(gcbh))
      mask TypeOptions Ts:
      | Angle/Integrator with
      | Wrapped State
      | (Discrete or Continuous)/Ts | PI/Integrator
      | (Discrete or Continuous)/Ts | Moving Average
      | (Variable Frequency)/Ts | Low-Pass Filter
      | (Discrete or Continuous)/Ts
      mask DialogControl Kp_LF Prompt: Loop filter proportional gain
      mask DialogControl Ki_LF Prompt: Loop filter integral gain
      mask DialogControl F0 Prompt: Initial frequency (Hz)
      mask DialogControl Theta0 Prompt: Initial phase angle (rad)
      mask DialogControl Ts Prompt: Sample time (-1 for inherited)
      mask Display: ee.mask.drawThreePhaseSinusoidalMeasurementPLL;
  Terminator : Terminator
  Terminator1 : Terminator
  abc1 : InportShadow
  mag : Outport
  freq : Outport  Port=2
  angle : Outport  Port=3
  Vd : Outport  Port=4
  Vq : Outport  Port=5
  Id : Outport  Port=6
  Iq : Outport  Port=7
  wires:
  Demux/3 -> Terminator/1
  Park Transform/1 -> Demux/1
  Demux/1 -> Vd/1
  Demux/2 -> Vq/1
  "Sinusoidal Measurement (PLL, Three-Phase)1"/3(mag) -> mag/1
  "Sinusoidal Measurement (PLL, Three-Phase)1"/2(angle) -> angle/1, Park Transform/2, Park Transform1/2
  Ig/1 -> Park Transform1/1
  Demux1/2 -> Iq/1
  Park Transform1/1 -> Demux1/1
  Demux1/1 -> Id/1
  Demux1/3 -> Terminator1/1
  abc1/1 -> Park Transform/1
  abc/1 -> "Sinusoidal Measurement (PLL, Three-Phase)1"/1(abc)
  "Sinusoidal Measurement (PLL, Three-Phase)1"/1(freq) -> freq/1

== system AdmittanceScanPRBS/Renewable Plant/PV Plant ==
  Vbus : Inport
  100 MWp PV Park : Subsystem
      settings: PortSchema="{\"entries\":[{\"content\":{\"sides\":[{\"content\":{\"connectorIds\":[\"Out1\",\"In1\",\"LConn1\"]},\"type\":\"ConnectorPlacement.EquallySpacedRectSide\",\"uuid\":\"343ce997-9cac-43fa-9216-298045fd67dd\"},{\"content\":{\"connectorIds\":[\"In2\"],\"side\":\"RIGHT\"},\"type\":\"ConnectorPlacement.EquallySpacedRectSide\",\"uuid\":\"419648e9-cc51-43b2-af12-d3f937f2b6d1\"},{\"content\":{\"side\":\"TOP\"},\"type\":\"ConnectorPlacement.EquallySpacedRectSide\",\"uuid\":\"296a2476-614b-49ee-a38a-605419a1856a\"},{\"content\":{\"side\":\"BOTTOM\"},\"type\":\"ConnectorPlacement.EquallySpacedRectSide\",\"uuid\":\"1a94dbbe-b4b3-4e2f-8128-897afc680bd0\"}]},\"type\":\"ConnectorPlacement.EquallySpacedConnector\",\"uuid\":\"83a42d0e-456a-4e37-b942-9ac5d756f0ba\"}],\"packageUris\":[\"http://schema.mathworks.com/mf0/Connector/R2020b\"],\"version\":\"1.0\"}"
      mask Display: image('$imagefile'); % Use "Edit Image" on toolstrip to change.
  60 MWhr Battery Energy Storage : Subsystem  mask{LabelModeActiveChoice1=BESSGridSupporting}
      mask prompts: LabelModeActiveChoice1 "Choose BESS Controller"
      settings: PortSchema="{\"entries\":[{\"content\":{\"sides\":[{\"content\":{\"connectorIds\":[\"In1\"]},\"type\":\"ConnectorPlacement.EquallySpacedRectSide\",\"uuid\":\"883e7b19-0e26-46af-952e-c8bc8ad7c7c8\"},{\"content\":{\"connectorIds\":[\"RConn1\",\"In2\",\"Out1\"],\"side\":\"RIGHT\"},\"type\":\"ConnectorPlacement.EquallySpacedRectSide\",\"uuid\":\"7a83414d-eb58-4460-b24e-307c8bde3358\"},{\"content\":{\"side\":\"TOP\"},\"type\":\"ConnectorPlacement.EquallySpacedRectSide\",\"uuid\":\"c6d607b7-7e86-4905-bc25-9c78b4ff15f7\"},{\"content\":{\"side\":\"BOTTOM\"},\"type\":\"ConnectorPlacement.EquallySpacedRectSide\",\"uuid\":\"e1bc4c26-6ec5-4df0-8f96-867ea0072814\"}]},\"type\":\"ConnectorPlacement.EquallySpacedConnector\",\"uuid\":\"ef2fc235-7b9f-436b-9d0c-7c76d6f36368\"}],\"packageUris\":[\"http://schema.mathworks.com/mf0/Connector/R2020b\"],\"version\":\"1.0\"}"
      mask TypeOptions LabelModeActiveChoice1: Variant Subsystem/LabelModeActiveChoice
      mask Display: image('$imagefile'); % Use "Edit Image" on toolstrip to change.
  Constant1 : Constant  Value=0
  Constant2 : Constant  Value=0
  "PV Plant Controller " : Subsystem
      settings: PortSchema="{\"entries\":[{\"content\":{\"sides\":[{\"content\":{\"connectorIds\":[\"In1\",\"Out1\"]},\"type\":\"ConnectorPlacement.EquallySpacedRectSide\",\"uuid\":\"4dd5c331-822d-4333-9dd3-7a69fe680142\"},{\"content\":{\"side\":\"RIGHT\"},\"type\":\"ConnectorPlacement.EquallySpacedRectSide\",\"uuid\":\"85556e6f-552b-436d-96c5-f50473e6eef2\"},{\"content\":{\"side\":\"TOP\"},\"type\":\"ConnectorPlacement.EquallySpacedRectSide\",\"uuid\":\"5ac869aa-0c48-488d-8d32-cb0a103032a5\"}]},\"type\":\"ConnectorPlacement.EquallySpacedConnector\",\"uuid\":\"1c77cf04-edee-41fe-a91f-465f3e8ec46b\"}],\"packageUris\":[\"http://schema.mathworks.com/mf0/Connector/R2020b\"],\"version\":\"1.0\"}"
      mask Display: image('$imagefile'); % Use "Edit Image" on toolstrip to change.
  Terminator : Terminator
  Terminator1 : Terminator
  abc : PMIOPort  Side=Right
  wires:
  "PV Plant Controller "/1(Q_ref) -> 100 MWp PV Park/2(Q_ref)
  Constant1/1 -> 100 MWp PV Park/1(LVRT_iq)
  Vbus/1 -> 60 MWhr Battery Energy Storage/1(Vbus), "PV Plant Controller "/1(Vbus)
  100 MWp PV Park/1(IPV) -> Terminator/1
  Constant2/1 -> 60 MWhr Battery Energy Storage/2(LVRT_iq)
  60 MWhr Battery Energy Storage/1(Bat) -> Terminator1/1
  connections:
  abc/RConn1 -- 60 MWhr Battery Energy Storage/RConn1 -- 100 MWp PV Park/LConn1
